simulink model "State_Observer_Design"  (R2020b)
settings: Solver=VariableStepAuto  StartTime=0.0  StopTime=10.0  RelTol=1e-3
settings Model: Creator=24365  LastModifiedBy=24365

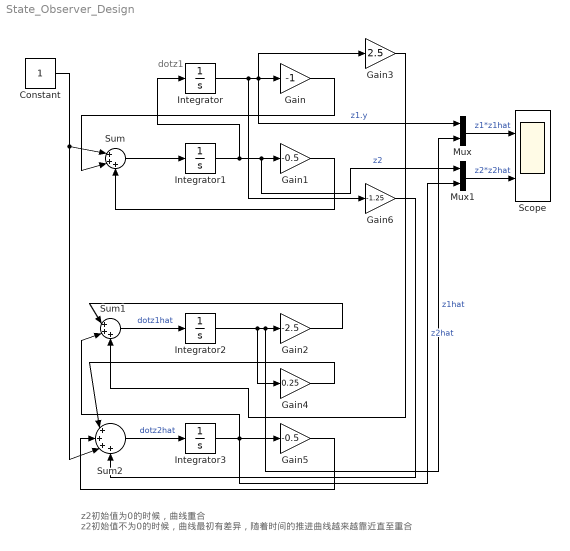
== system State_Observer_Design ==
  note: z2初始值为0的时候，曲线重合
      | z2初始值不为0的时候，曲线最初有差异，随着时间的推进曲线越来越靠近直至重合
  note: dotz1
  Constant : Constant
  Gain : Gain  Gain=-1
  Gain1 : Gain  Gain=-0.5
  Gain2 : Gain  Gain=-2.5
  Gain3 : Gain  Gain=2.5
  Gain4 : Gain  Gain=0.25
  Gain5 : Gain  Gain=-0.5
  Gain6 : Gain  Gain=-1.25
  Integrator : Integrator
  Integrator1 : Integrator
  Integrator2 : Integrator
  Integrator3 : Integrator  InitialCondition=1
  Mux : Mux  Inputs=2
  Mux1 : Mux  Inputs=2
  Scope : Scope  NumInputPorts=2
  Sum : Sum  Inputs=|+++
  Sum1 : Sum  Inputs=|+++
  Sum2 : Sum  Inputs=|++++
  wires:
  Integrator1/1 -> Mux1/1, Gain1/1, Integrator/1  "z2"
  Sum/1 -> Integrator1/1
  Integrator/1 -> Gain6/1, Mux/1, Gain3/1, Gain/1  "z1.y"
  Gain1/1 -> Sum/3
  Gain/1 -> Sum/2
  Constant/1 -> Sum2/3, Sum/1
  Integrator2/1 -> Gain4/1, Mux/2, Gain2/1  "z1hat"
  Sum1/1 -> Integrator2/1  "dotz1hat"
  Integrator3/1 -> Mux1/2, Gain5/1, Sum1/2  "z2hat"
  Sum2/1 -> Integrator3/1  "dotz2hat"
  Gain2/1 -> Sum1/1
  Gain3/1 -> Sum1/3
  Gain4/1 -> Sum2/1
  Gain5/1 -> Sum2/2
  Gain6/1 -> Sum2/4
  Mux/1 -> Scope/1  "z1*z1hat"
  Mux1/1 -> Scope/2  "z2*z2hat"
